simulink subsystem "LuenbergerObserver"  (R2023b)
settings: Solver=VariableStepAuto  StartTime=0.0  StopTime=10.0  RelTol=1e-3
values from neighbouring files (symbols this model uses):
  a1 = 83820765.49    [params_aaa_elb.mat]
  b1 = 0.0647    [params_aaa_elb.mat]
  cm2m = 0.01    [params_aaa_elb.mat]
  f1 = 1170    [params_aaa_elb.mat]
  f2 = -880    [params_aaa_elb.mat]
  g = 9.816    [params_aaa_elb.mat]
  g1 = -6.51    [params_aaa_elb.mat]
  g2 = 3.66    [params_aaa_elb.mat]
  h1 = 1.53e-05    [params_aaa_elb.mat]
  h2 = 2e-05    [params_aaa_elb.mat]
  m = 0.1203    [params_aaa_elb.mat]
  N = 4    [params_aaa_elb.mat]
  SatLimLower = -14000    [params_aaa_elb.mat]
  SatLimUpper = 14000    [params_aaa_elb.mat]
  Ts = 0.00442    [params_aaa_elb.mat]
undefined symbols (not defined in the file or in its folder): L2, L3, sine_A, sine_f, u10_sine
libraries: simulink x1
settings Model: Creator=amaln  LastModifiedBy=amaln

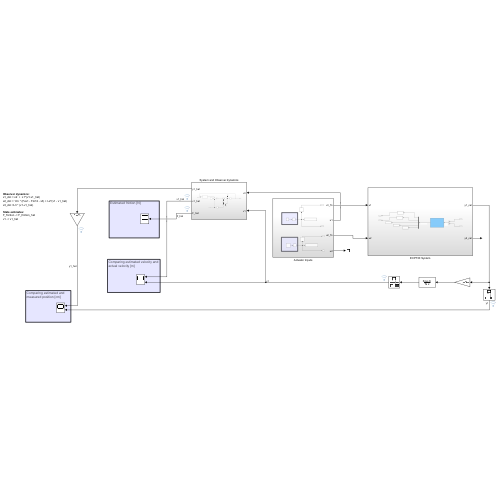
[thumbnail: Simulink's stored preview of the top-level diagram]
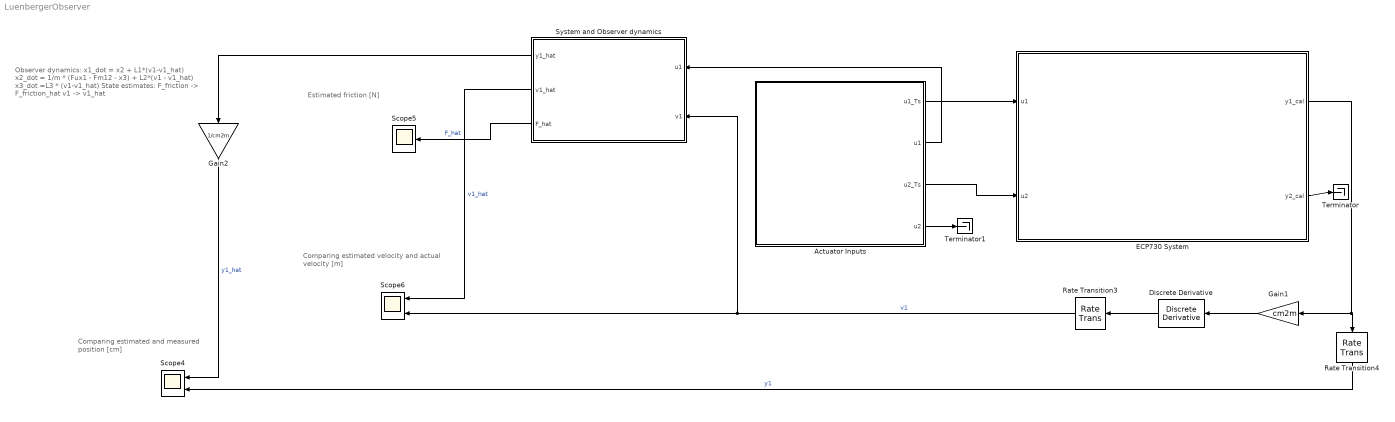
== system LuenbergerObserver ==
  note: Estimated friction [N]
  note: Comparing estimated velocity and
      | actual velocity [m]
  note: Comparing estimated and
      | measured position [cm]
  note: Observer dynamics:
      | x1_dot = x2 + L1*(v1-v1_hat)
      | x2_dot = 1/m * (Fux1 - Fm12 - x3) + L2*(v1 - v1_hat)
      | x3_dot =L3 * (v1-v1_hat)
      |
      | State estimates:
      | F_friction -> F_friction_hat
      | v1 -> v1_hat
  Actuator Inputs : Subsystem
  Discrete Derivative : simulink/Discrete/Discrete Derivative  gainval=1.0  ICPrevScaledInput=0.0  OutMin=[]  OutMax=[]  OutDataType=fixdt(1, 16)  OutScaling=2^-10  DoSatur=off
  ECP730 System : Subsystem
  Gain1 : Gain  Gain=cm2m
  Gain2 : Gain  Gain=1/cm2m
  Rate Transition3 : RateTransition  OutPortSampleTime=STEP_SIZE
  Rate Transition4 : RateTransition  OutPortSampleTime=STEP_SIZE
  Scope4 : Scope  NumInputPorts=2
  Scope5 : Scope
  Scope6 : Scope  NumInputPorts=2
  System and Observer dynamics : Subsystem
  Terminator : Terminator
  Terminator1 : Terminator
  wires:
  ECP730 System/2(y2_cal) -> Terminator/1
  Actuator Inputs/3(u2_Ts) -> ECP730 System/2(u2)
  Actuator Inputs/2(u1) -> System and Observer dynamics/1(u1)
  Actuator Inputs/1(u1_Ts) -> ECP730 System/1(u1)
  ECP730 System/1(y1_cal) -> Rate Transition4/1, Gain1/1
  Discrete Derivative/1 -> Rate Transition3/1
  System and Observer dynamics/1(y1_hat) -> Gain2/1
  System and Observer dynamics/3(F_hat) -> Scope5/1  "F_hat"
  System and Observer dynamics/2(v1_hat) -> Scope6/1  "v1_hat"
  Gain2/1 -> Scope4/1  "y1_hat"
  Gain1/1 -> Discrete Derivative/1
  Rate Transition3/1 -> System and Observer dynamics/2(v1), Scope6/2  "v1"
  Rate Transition4/1 -> Scope4/2  "y1"
  Actuator Inputs/4(u2) -> Terminator1/1

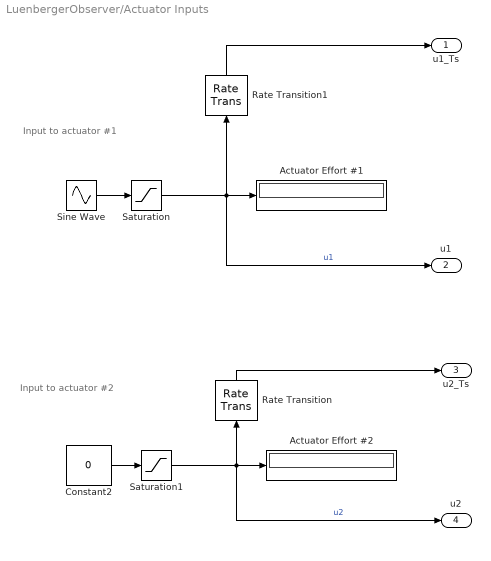
== system LuenbergerObserver/Actuator Inputs ==
  note: Input to actuator #1
  note: Input to actuator #2
  Actuator Effort #1 : Display
  Actuator Effort #2 : Display
  Constant2 : Constant  Value=0
  Rate Transition : RateTransition  OutPortSampleTime=Ts
  Rate Transition1 : RateTransition  OutPortSampleTime=Ts
  Saturation : Saturate  UpperLimit=SatLimUpper  LowerLimit=SatLimLower
  Saturation1 : Saturate  UpperLimit=SatLimUpper  LowerLimit=SatLimLower
  Sine Wave : Sin  Amplitude=sine_A  Bias=u10_sine  Frequency=2*pi*sine_f  SampleTime=0
  u1_Ts : Outport
  u1 : Outport  Port=2
  u2_Ts : Outport  Port=3
  u2 : Outport  Port=4
  wires:
  Saturation/1 -> Rate Transition1/1, Actuator Effort #1/1, u1/1  "u1"
  Constant2/1 -> Saturation1/1
  Sine Wave/1 -> Saturation/1
  Rate Transition1/1 -> u1_Ts/1
  Rate Transition/1 -> u2_Ts/1
  Saturation1/1 -> Actuator Effort #2/1, Rate Transition/1, u2/1  "u2"

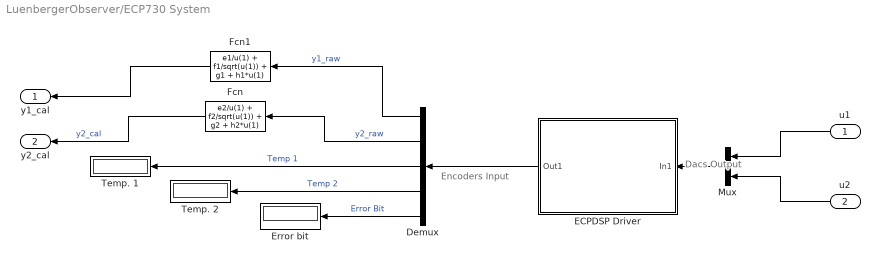
== system LuenbergerObserver/ECP730 System ==
  note: Encoders Input
  note: Dacs
      | Output
  u1 : Inport
  u2 : Inport  Port=2
  Demux : Demux  Outputs=5
      settings: DisplayOption=none
  ECPDSP Driver : Subsystem  mask{BaseAddr='0x3F00', STime=Ts, TimeOutPer=500, HWAccess=on}
      mask prompts: BaseAddr "Base I/O Address"; STime "Sample Time (Sec)"; TimeOutPer "Timeout Period (500 ~ 2000)"; HWAccess "Hardware Access"
      mask Display: color('black');disp('ECPDSP Driver\n upto\n 4 Encs(ADC Channels)\n and 2 Dacs')
  "Error bit " : Display
  Fcn : Fcn  Expr=e2/u(1) + f2/sqrt(u(1)) + g2 + h2*u(1)
  Fcn1 : Fcn  Expr=e1/u(1) + f1/sqrt(u(1)) + g1 + h1*u(1)
  Mux : Mux  Inputs=2
  Temp. 1 : Display
  Temp. 2 : Display
  y1_cal : Outport
  y2_cal : Outport  Port=2
  wires:
  u2/1 -> Mux/2
  Demux/1 -> Fcn1/1  "y1_raw"
  u1/1 -> Mux/1
  Mux/1 -> ECPDSP Driver/1(In1)
  Demux/3 -> Temp. 1/1  "Temp 1"
  ECPDSP Driver/1(Out1) -> Demux/1
  Demux/5 -> "Error bit "/1  "Error Bit"
  Demux/2 -> Fcn/1  "y2_raw"
  Demux/4 -> Temp. 2/1  "Temp 2"
  Fcn/1 -> y2_cal/1  "y2_cal"
  Fcn1/1 -> y1_cal/1

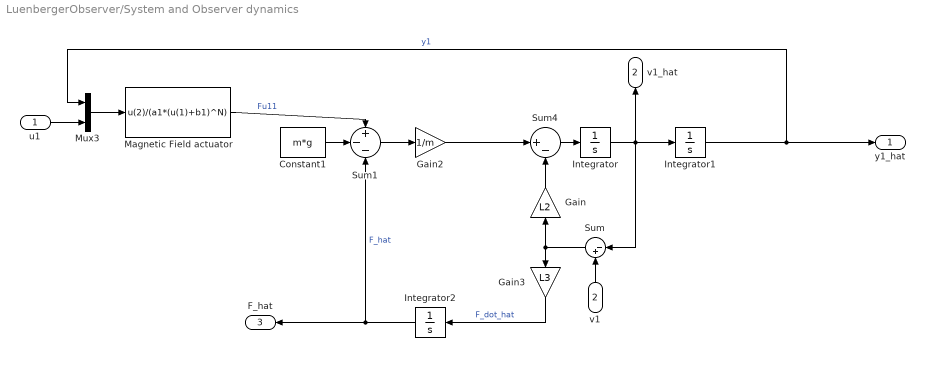
== system LuenbergerObserver/System and Observer dynamics ==
  u1 : Inport
  v1 : Inport  Port=2
  Constant1 : Constant  Value=m*g
  Gain : Gain  Gain=L2
  Gain2 : Gain  Gain=1/m
  Gain3 : Gain  Gain=L3
  Integrator : Integrator
  Integrator1 : Integrator
  Integrator2 : Integrator
  Magnetic Field actuator : Fcn  Expr=u(2)/(a1*(u(1)+b1)^N)
  Mux3 : Mux  Inputs=2
  Sum : Sum  Inputs=|-+
  Sum1 : Sum  Inputs=+--
  Sum4 : Sum  Inputs=|+-
  y1_hat : Outport  VectorParamsAs1DForOutWhenUnconnected=off
  v1_hat : Outport  Port=2  VectorParamsAs1DForOutWhenUnconnected=off
  F_hat : Outport  Port=3  VectorParamsAs1DForOutWhenUnconnected=off
  wires:
  Constant1/1 -> Sum1/2
  Sum1/1 -> Gain2/1
  Magnetic Field actuator/1 -> Sum1/1  "Fu11"
  Mux3/1 -> Magnetic Field actuator/1
  Integrator1/1 -> y1_hat/1, Mux3/1  "y1"
  v1/1 -> Sum/2
  Gain2/1 -> Sum4/1
  Sum4/1 -> Integrator/1
  Sum/1 -> Gain/1, Gain3/1
  Gain/1 -> Sum4/2
  u1/1 -> Mux3/2
  Gain3/1 -> Integrator2/1  "F_dot_hat"
  Integrator2/1 -> Sum1/3, F_hat/1  "F_hat"
  Integrator/1 -> Integrator1/1, Sum/1, v1_hat/1

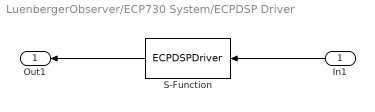
== system LuenbergerObserver/ECP730 System/ECPDSP Driver ==
  In1 : Inport
  S-Function : S-Function  FunctionName=ECPDSPDriver  Parameters=BaseAddr,STime,TimeOutPer,HWAccess  SFunctionDeploymentMode=off  EnableBusSupport=off
  Out1 : Outport  VectorParamsAs1DForOutWhenUnconnected=off
  wires:
  In1/1 -> S-Function/1
  S-Function/1 -> Out1/1
